simulink model "test_1"  (R2018b)
settings: Solver=VariableStepAuto  StartTime=0.0  StopTime=10.0  RelTol=1e-3
undefined symbols (not defined in the file): sigbuilder_block
settings Model: Creator=michask  LastModifiedBy=michask

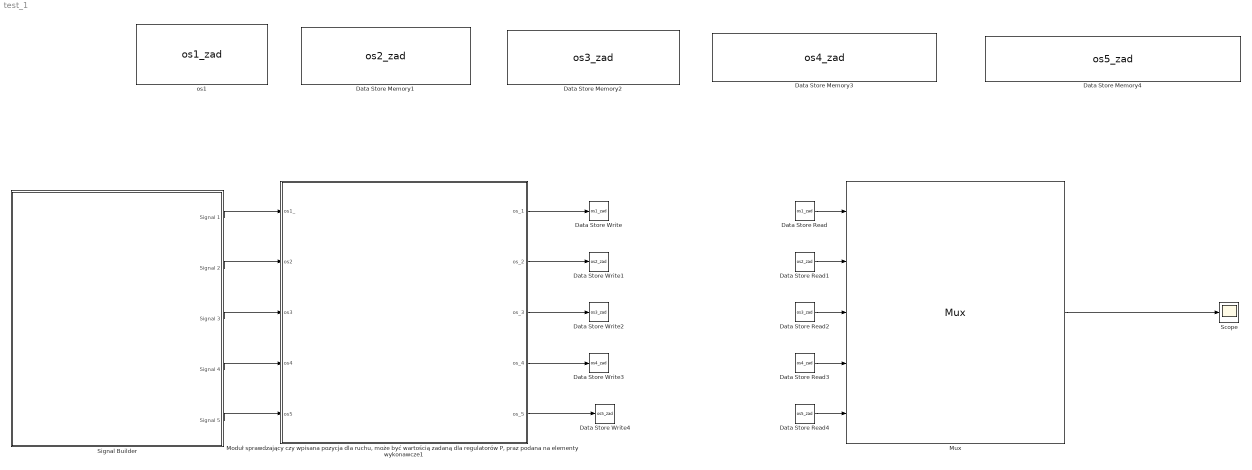
== system test_1 ==
  Data Store Memory1 : DataStoreMemory  DataStoreName=os2_zad  ReadBeforeWriteMsg=warning  WriteAfterWriteMsg=warning  WriteAfterReadMsg=warning  ShowAdditionalParam=off
  Data Store Memory2 : DataStoreMemory  DataStoreName=os3_zad  ReadBeforeWriteMsg=warning  WriteAfterWriteMsg=warning  WriteAfterReadMsg=warning  ShowAdditionalParam=off
  Data Store Memory3 : DataStoreMemory  DataStoreName=os4_zad  ReadBeforeWriteMsg=warning  WriteAfterWriteMsg=warning  WriteAfterReadMsg=warning  ShowAdditionalParam=off
  Data Store Memory4 : DataStoreMemory  DataStoreName=os5_zad  ReadBeforeWriteMsg=warning  WriteAfterWriteMsg=warning  WriteAfterReadMsg=warning  ShowAdditionalParam=off
  Data Store Read : DataStoreRead  DataStoreName=os1_zad
  Data Store Read1 : DataStoreRead  DataStoreName=os2_zad
  Data Store Read2 : DataStoreRead  DataStoreName=os3_zad
  Data Store Read3 : DataStoreRead  DataStoreName=os4_zad
  Data Store Read4 : DataStoreRead  DataStoreName=os5_zad
  Data Store Write : DataStoreWrite  DataStoreName=os1_zad
  Data Store Write1 : DataStoreWrite  DataStoreName=os2_zad
  Data Store Write2 : DataStoreWrite  DataStoreName=os3_zad
  Data Store Write3 : DataStoreWrite  DataStoreName=os4_zad
  Data Store Write4 : DataStoreWrite  DataStoreName=os5_zad
  "Moduł sprawdzający czy wpisana pozycja dla ruchu, może być wartością zadaną dla regulatorów P, praz podana na elementy wykonawcze1" : Subsystem
  Mux : Mux  Inputs=5
  Scope : Scope
  Signal Builder : Subsystem  Tag=STV Subsys  LoadFcn=sigbuilder_block('load');  StartFcn=sigbuilder_block('start');  StopFcn=sigbuilder_block('stop');  ClipboardFcn=sigbuilder_block('clipboard');  mask(Sigbuilder block){tuvar=[0:10]}
      mask help: Simulink:masks:SigbuilderBlock_MD
      mask init:
      | if ~strcmp(get_param(bdroot(gcbh),'SimulationStatus'),'stopped') tuvar = sigbuilder_block('maskInit'); end
      settings: CopyFcn=sigbuilder_block('copy');  DeleteFcn=sigbuilder_block('delete');  ModelCloseFcn=sigbuilder_block('modelClose');  PreSaveFcn=sigbuilder_block('preSave');  PauseFcn=sigbuilder_block('pause');  ContinueFcn=sigbuilder_block('continue');  NameChangeFcn=sigbuilder_block('namechange');  OpenFcn=sigbuilder_block('open',[5.4 30 1141.2 522.6 ]);  CloseFcn=sigbuilder_block('close');
      mask Display: plot(0, 0, 100, 100,[2, 2, 32, 32, 2], [68, 8, 8, 68, 68],[32, 2], [38, 38], [32, 19, 2],[53, 60, 44], [32, 17, 17, 2],[16, 16, 31, 31]);txt = getActiveGroup(gcbh);text(2, 100, txt,'verticalAlignment', 'top');
  os1 : DataStoreMemory  DataStoreName=os1_zad  ReadBeforeWriteMsg=warning  WriteAfterWriteMsg=warning  WriteAfterReadMsg=warning  ShowAdditionalParam=off
  wires:
  Mux/1 -> Scope/1
  Data Store Read1/1 -> Mux/2
  Data Store Read2/1 -> Mux/3
  Data Store Read/1 -> Mux/1
  Data Store Read3/1 -> Mux/4
  Data Store Read4/1 -> Mux/5
  "Moduł sprawdzający czy wpisana pozycja dla ruchu, może być wartością zadaną dla regulatorów P, praz podana na elementy wykonawcze1"/5(os_5) -> Data Store Write4/1
  "Moduł sprawdzający czy wpisana pozycja dla ruchu, może być wartością zadaną dla regulatorów P, praz podana na elementy wykonawcze1"/4(os_4) -> Data Store Write3/1
  "Moduł sprawdzający czy wpisana pozycja dla ruchu, może być wartością zadaną dla regulatorów P, praz podana na elementy wykonawcze1"/3(os_3) -> Data Store Write2/1
  "Moduł sprawdzający czy wpisana pozycja dla ruchu, może być wartością zadaną dla regulatorów P, praz podana na elementy wykonawcze1"/2(os_2) -> Data Store Write1/1
  "Moduł sprawdzający czy wpisana pozycja dla ruchu, może być wartością zadaną dla regulatorów P, praz podana na elementy wykonawcze1"/1(os_1) -> Data Store Write/1
  Signal Builder/1(Signal 1) -> "Moduł sprawdzający czy wpisana pozycja dla ruchu, może być wartością zadaną dla regulatorów P, praz podana na elementy wykonawcze1"/1(os1_)
  Signal Builder/2(Signal 2) -> "Moduł sprawdzający czy wpisana pozycja dla ruchu, może być wartością zadaną dla regulatorów P, praz podana na elementy wykonawcze1"/2(os2)
  Signal Builder/3(Signal 3) -> "Moduł sprawdzający czy wpisana pozycja dla ruchu, może być wartością zadaną dla regulatorów P, praz podana na elementy wykonawcze1"/3(os3)
  Signal Builder/4(Signal 4) -> "Moduł sprawdzający czy wpisana pozycja dla ruchu, może być wartością zadaną dla regulatorów P, praz podana na elementy wykonawcze1"/4(os4)
  Signal Builder/5(Signal 5) -> "Moduł sprawdzający czy wpisana pozycja dla ruchu, może być wartością zadaną dla regulatorów P, praz podana na elementy wykonawcze1"/5(os5)

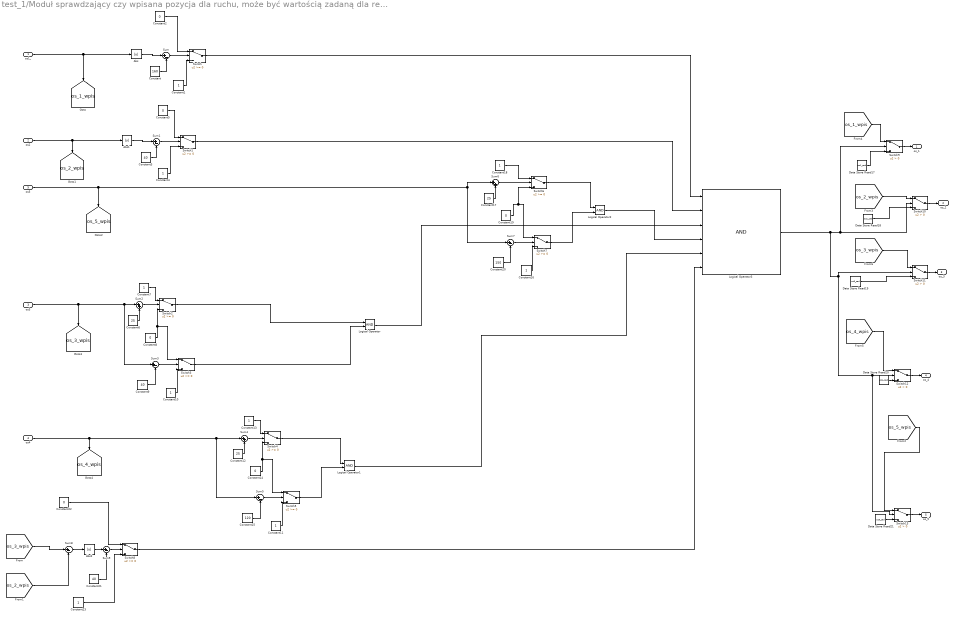
== system test_1/Moduł sprawdzający czy wpisana pozycja dla ruchu, może być wartością zadaną dla regulatorów P, praz podana na elementy wykonawcze1 ==
  os1_ : Inport
  os2 : Inport  Port=2
  os3 : Inport  Port=3
  os4 : Inport  Port=4
  os5 : Inport  Port=5
  Abs : Abs
  Abs1 : Abs
  Abs2 : Abs
  Constant : Constant  Value=160
  Constant{1,4,7,10..11,13,16,18,23} (9 alike) : Constant
  Constant12 : Constant  Value=25
  Constant{2,5,8,14,19,22} (6 alike) : Constant  Value=0
  Constant15 : Constant  Value=120
  Constant17 : Constant  Value=25
  Constant20 : Constant  Value=150
  Constant21 : Constant  Value=40
  Constant3 : Constant  Value=40
  Constant6 : Constant  Value=25
  Constant9 : Constant  Value=40
  Data Store Read17 : DataStoreRead  DataStoreName=os1_zad
  Data Store Read18 : DataStoreRead  DataStoreName=os2_zad
  Data Store Read19 : DataStoreRead  DataStoreName=os3_zad
  Data Store Read20 : DataStoreRead  DataStoreName=os4_zad
  Data Store Read21 : DataStoreRead  DataStoreName=os5_zad
  Logical Operator : Logic  AllPortsSameDT=off
  Logical Operator1 : Logic  AllPortsSameDT=off
  Logical Operator2 : Logic  AllPortsSameDT=off
  Logical Operator3 : Logic  Inputs=6  AllPortsSameDT=off
  Sum{,1,3,5,7..9} (7 alike) : Sum  Inputs=|+-
  Sum2 : Sum  Inputs=|++
  Sum4 : Sum  Inputs=|++
  Sum6 : Sum  Inputs=|++
  Switch{,1..8} (9 alike) : Switch
  Switch{9..13} (5 alike) : Switch  Criteria=u2 > Threshold
  os_1 : Outport
  os_2 : Outport  Port=2
  os_3 : Outport  Port=3
  os_4 : Outport  Port=4
  os_5 : Outport  Port=5
  tag scope: os_1_wpis=global, os_2_wpis=global, os_3_wpis=global, os_4_wpis=global, os_5_wpis=global
  wires:
  Constant18/1 -> Switch6/1
  Data Store Read19/1 -> Switch11/3
  [os_3_wpis] -> Switch11/1
  os3/1 -> Sum3/1, Sum2/1, [os_3_wpis]
  Sum2/1 -> Switch2/2
  Switch8/1 -> Logical Operator3/6
  Abs/1 -> Sum/1
  Abs2/1 -> Sum9/1
  os2/1 -> Abs1/1, [os_2_wpis]
  Switch7/1 -> Logical Operator2/2
  Logical Operator/1 -> Logical Operator3/3
  Constant21/1 -> Sum9/2
  Constant20/1 -> Sum7/2
  Constant10/1 -> Switch3/3
  Switch5/1 -> Logical Operator1/2
  Constant3/1 -> Sum1/2
  [os_2_wpis] -> Switch10/1
  Sum6/1 -> Switch6/2
  Constant19/1 -> Switch7/1, Switch6/3
  Sum8/1 -> Abs2/1
  Constant16/1 -> Switch7/3
  Constant1/1 -> Switch/3
  Logical Operator2/1 -> Logical Operator3/4
  Sum/1 -> Switch/2
  os5/1 -> [os_5_wpis], Sum6/1, Sum7/1
  Constant7/1 -> Switch2/1
  Constant14/1 -> Switch5/1, Switch4/3
  Logical Operator1/1 -> Logical Operator3/5
  [os_5_wpis] -> Switch13/1
  Switch6/1 -> Logical Operator2/1
  [os_4_wpis] -> Switch12/1
  Sum7/1 -> Switch7/2
  Data Store Read20/1 -> Switch12/3
  Switch1/1 -> Logical Operator3/2
  Constant8/1 -> Switch3/1, Switch2/3
  Abs1/1 -> Sum1/1
  [os_1_wpis] -> Switch9/1
  Constant9/1 -> Sum3/2
  Constant6/1 -> Sum2/2
  Constant/1 -> Sum/2
  Switch/1 -> Logical Operator3/1
  Data Store Read17/1 -> Switch9/3
  Data Store Read21/1 -> Switch13/3
  Data Store Read18/1 -> Switch10/3
  Switch4/1 -> Logical Operator1/1
  Sum5/1 -> Switch5/2
  Constant5/1 -> Switch1/1
  Logical Operator3/1 -> Switch13/2, Switch12/2, Switch11/2, Switch10/2, Switch9/2
  Constant22/1 -> Switch8/1
  Constant4/1 -> Switch1/3
  Constant2/1 -> Switch/1
  Constant13/1 -> Switch4/1
  Sum3/1 -> Switch3/2
  Switch3/1 -> Logical Operator/2
  Sum4/1 -> Switch4/2
  os4/1 -> [os_4_wpis], Sum4/1, Sum5/1
  Switch2/1 -> Logical Operator/1
  Constant11/1 -> Switch5/3
  Constant17/1 -> Sum6/2
  Constant12/1 -> Sum4/2
  Constant15/1 -> Sum5/2
  Sum9/1 -> Switch8/2
  Constant23/1 -> Switch8/3
  Sum1/1 -> Switch1/2
  os1_/1 -> [os_1_wpis], Abs/1
  Switch9/1 -> os_1/1
  Switch10/1 -> os_2/1
  Switch11/1 -> os_3/1
  Switch12/1 -> os_4/1
  Switch13/1 -> os_5/1
  [os_3_wpis] -> Sum8/1
  [os_2_wpis] -> Sum8/2

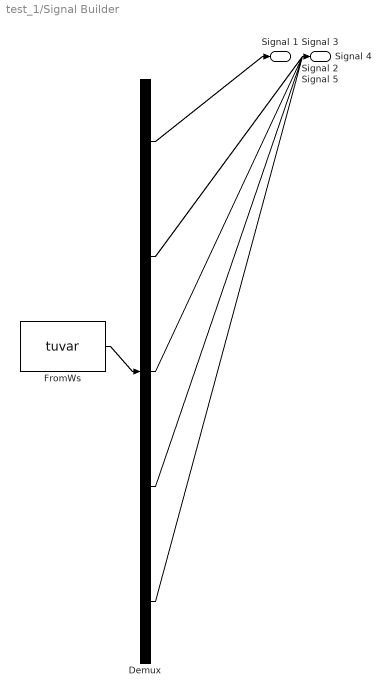
== system test_1/Signal Builder ==
  Demux : Demux  Tag=STV Demux  Outputs=5
  FromWs : FromWorkspace  Tag=STV FromWs  VariableName=tuvar  SampleTime=0
      SigBuilderData=|
      | common.afterFinalStr = 'Extrapolate'
      | common.sampleTime = 0
      | dataSet(1).timeRange = [0 10]
      | dataSet(1).name = 'Group 1'
      | dataSet(2).timeRange = [0 10]
      | dataSet(2).name = 'Group 2'
      | dataSet(3).timeRange = [0 10]
      | dataSet(3).name = 'Group 3'
      | sbobj.Groups(1).Name = 'Group 1'
      | sbobj.Groups(1).Signals(1).Name = 'Signal 1'
      | sbobj.Groups(1).Signals(1).XData = [0 1 2 3 4 4 5 5.5 6 10]
      | sbobj.Groups(1).Signals(1).YData = [0 -150 2 30 50 45 195 200 200 6]
      | sbobj.Groups(1).Signals(2).Name = 'Signal 2'
      | sbobj.Groups(1).Signals(2).XData = [0 1 2 3 4 5 10]
      | sbobj.Groups(1).Signals(2).YData = [0 -35 0 10 -40 0 0]
      | sbobj.Groups(1).Signals(3).Name = 'Signal 3'
      | sbobj.Groups(1).Signals(3).XData = [0 1 2 3 4 5 10]
      | sbobj.Groups(1).Signals(3).YData = [0 -20 0 10 5 8 5]
      | sbobj.Groups(1).Signals(4).Name = 'Signal 4'
      | sbobj.Groups(1).Signals(4).XData = [0 1 2 3 4 5 10]
      | sbobj.Groups(1).Signals(4).YData = [0 -20 0 10 15 7 15]
      | sbobj.Groups(1).Signals(5).Name = 'Signal 5'
      | sbobj.Groups(1).Signals(5).XData = [0 1 2 3 4 5 10]
      | sbobj.Groups(1).Signals(5).YData = [0 -20 6 10 15 5 15]
      | sbobj.Groups(2).Name = 'Group 2'
      | sbobj.Groups(2).Signals(1).Name = 'Signal 1'
      | sbobj.Groups(2).Signals(1).XData = [0 1 2 3 4 4 5 5.5 6 10]
      | sbobj.Groups(2).Signals(1).YData = [0 380 350 360 330 45 350 370 -300 6]
      | sbobj.Groups(2).Signals(2).Name = 'Signal 2'
      | sbobj.Groups(2).Signals(2).XData = [0 1 2 3 4 5 10]
      | sbobj.Groups(2).Signals(2).YData = [0 -35 0 10 -40 0 0]
      | sbobj.Groups(2).Signals(3).Name = 'Signal 3'
      | sbobj.Groups(2).Signals(3).XData = [0 1 2 3 4 5 10]
      | sbobj.Groups(2).Signals(3).YData = [0 -20 0 10 5 8 5]
      | sbobj.Groups(2).Signals(4).Name = 'Signal 4'
      | sbobj.Groups(2).Signals(4).XData = [0 1 2 3 4 5 10]
      | sbobj.Groups(2).Signals(4).YData = [0 -20 0 10 15 7 15]
      | sbobj.Groups(2).Signals(5).Name = 'Signal 5'
      | sbobj.Groups(2).Signals(5).XData = [0 1 2 3 4 5 10]
      | sbobj.Groups(2).Signals(5).YData = [0 -20 6 10 15 5 15]
      | sbobj.Groups(3).Name = 'Group 3'
      | sbobj.Groups(3).Signals(1).Name = 'Signal 1'
      | sbobj.Groups(3).Signals(1).XData = [0 2 2 3 4 4 5 5.5 6 10]
      | sbobj.Groups(3).Signals(1).YData = [0 0 30 40 50 45 180 180 50 6]
      | sbobj.Groups(3).Signals(2).Name = 'Signal 2'
      | sbobj.Groups(3).Signals(2).XData = [0 1 2 3 4 5 10]
      | sbobj.Groups(3).Signals(2).YData = [0 -35 0 -40 -40 -39 0]
      | sbobj.Groups(3).Signals(3).Name = 'Signal 3'
      | sbobj.Groups(3).Signals(3).XData = [0 1 2 3 4 5 10]
      | sbobj.Groups(3).Signals(3).YData = [0 -20 0 10 5 8 5]
      | sbobj.Groups(3).Signals(4).Name = 'Signal 4'
      | sbobj.Groups(3).Signals(4).XData = [0 1 2 3 4 5 10]
      | sbobj.Groups(3).Signals(4).YData = [0 -20 0 -13 15 7 15]
      | sbobj.Groups(3).Signals(5).Name = 'Signal 5'
      | sbobj.Groups(3).Signals(5).XData = [0 1 2 3 4 5 10]
      | sbobj.Groups(3).Signals(5).YData = [0 -20 6 10 -10 5 15]
  Signal 1 : Outport  Tag=STV Outport
  Signal 2 : Outport  Tag=STV Outport  Port=2
  Signal 3 : Outport  Tag=STV Outport  Port=3
  Signal 4 : Outport  Tag=STV Outport  Port=4
  Signal 5 : Outport  Tag=STV Outport  Port=5
  wires:
  Demux/1 -> Signal 1/1
  Demux/2 -> Signal 2/1
  Demux/3 -> Signal 3/1
  Demux/4 -> Signal 4/1
  Demux/5 -> Signal 5/1
  FromWs/1 -> Demux/1
